simulink model "Outputswitch_Model"  (R2024b)
settings: Solver=VariableStepAuto  StartTime=0.0  StopTime=10.0  RelTol=1e-3
libraries: NSA_DEVS_SINKS x4, NSA_DEVS_SOURCES x2, NSA_DEVS_ROUTING x1
settings Model: Creator=david  LastModifiedBy=peter
settings RTWCC: GPUComputeCapability=3.5

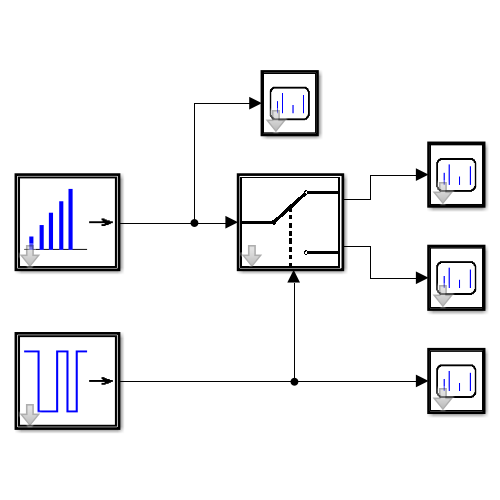
[thumbnail: Simulink's stored preview of the top-level diagram]
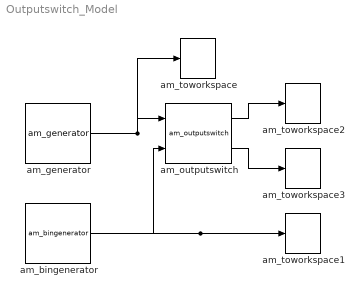
== system Outputswitch_Model ==
  am_bingenerator : NSA_DEVS_SOURCES/am_bingenerator  z0=true  tVec=[3, 8, 9, 10, 12, 17]  tau=[0,1]  debug=0
      settings: SourceProductName=Sources
  am_generator : NSA_DEVS_SOURCES/am_generator  tG=1  n0=1  nG=100  tD=[0,2]  debug=0
      settings: SourceProductName=Sources
  am_outputswitch : NSA_DEVS_ROUTING/am_outputswitch  port0=1  tau=[0,1]  debug=0
      settings: SourceProductName=Routing
  am_toworkspace : NSA_DEVS_SINKS/am_toworkspace  varname="\"genOut\""  t0=0  format="\"vector\""  tau=[0,5]  debug=0
      settings: SourceProductName=Sinks
  am_toworkspace1 : NSA_DEVS_SINKS/am_toworkspace  varname="\"vgenOut\""  t0=0  format="\"vector\""  tau=[0,5]  debug=0
      settings: SourceProductName=Sinks
  am_toworkspace2 : NSA_DEVS_SINKS/am_toworkspace  varname="\"sw1Out\""  t0=0  format="\"vector\""  tau=[0,5]  debug=0
      settings: SourceProductName=Sinks
  am_toworkspace3 : NSA_DEVS_SINKS/am_toworkspace  varname="\"sw2Out\""  t0=0  format="\"vector\""  tau=[0,5]  debug=0
      settings: SourceProductName=Sinks
  wires:
  am_generator/1 -> am_toworkspace/1, am_outputswitch/1
  am_bingenerator/1 -> am_outputswitch/2, am_toworkspace1/1
  am_outputswitch/1 -> am_toworkspace2/1
  am_outputswitch/2 -> am_toworkspace3/1
